simulink model "EPT"  (R2019b)
settings: Solver=FixedStepDiscrete  StartTime=0.0  StopTime=5  FixedStep=0.005  RelTol=1e-3  EnableMultiTasking=on
PreLoadFcn:
  | try, model_open; catch, disp('Error occurred while executing model pre-load callback: model_open.m'); disp('Please assure that the MATLAB working directory is set to the model directory before opening.'); end
InitFcn:
  | try, model_open; catch, end
undefined symbols (not defined in the file or in its folder): Bridge, GCM, H, ln, raptor_get_param_eval, raptor_get_safe_string, raptor_xcp_function
libraries: Raptor_lib x2810, simulink x374, hdlsllib x19
(part 18 of 45)

== system EPT/Foreground_TimeBase_5ms/CAN/CAN3_exec/DCDC/DCDC_RX_0x180XF45D  ==
  Trigger : TriggerPort  VariantControl=Variant  PortDimensions=1
  Constant : Constant  Value=0.1
  Constant1 : Constant  Value=-40
  Constant2 : Constant
  Convert_Byte2Data1 : Subsystem
  Convert_Byte2Data2 : Subsystem
  Convert_Byte2Data3 : Subsystem
  Demux : Demux  Outputs=8
  raptor_can_rxmsg : Raptor_lib/CAN/raptor_can_rxmsg  Commented=on  canDefinition=struct('dbcFile', 'DCDC_TDY_1Y_108_12 _V07.dbc','message', 'DCDC2EPT','comment', '','signals', {{'Output_Voltage','Output_Current','Internal_Temp','Status'}},'enabled', [ 1 1 1 1;],'canBus', '''CAN3''','messageID', [ 403174613;],'idMask', [ 536870911;],'payloadMask', [],'payloadValue', [],'period', [ 0;],'mailbox', '''''','queueSize', [ 1;],'label', [ 0;],'ver', [ 2;],'showID', [ 0;],'showRaw', [ 0;],'fill', [ 0;],'editID', [ 0;],'signalOrder', [ 2;])  canBus='CAN3'  mailbox=''  payloadMask=[]  payloadValue=[]  idMask=hex2dec('1FFFFFFF')  queueSize=1  showID=0  label=0  fill=0  id=403174613  showRaw=0  showAge=1  signalOrder=2  signalInfo={{struct('Name', 'Status','Startbit', [ 0;],'SignalSize', [ 8;],'ByteOrder', 'BigEndian','ValueType', 'UNSIGNED','Class', 'uint8','Signed', [ 0;],'Factor', [ 1;],'Offset', [ 0;],'Min', [ 0;],'Max', [ 0;],'Units', '','Comment', '','StartBit', [ 40;]),struct('Name', 'Output_Voltage','Startbit', [ 0;],'SignalSize', [ 16;],'ByteOrder', 'BigEndian','ValueType', 'UNSIGNED','Class', 'uint16','Signed', [ 0;],'Factor', [ 0.1;],'Offset', [ 0;],'Min', [ 0;],'Max', [ 0;],'Units', 'V','Comment', '','StartBit', [ 8;]),struct('Name', 'Output_Current','Startbit', [ 0;],'SignalSize', [ 16;],'ByteOrder', 'BigEndian','ValueType', 'UNSIGNED','Class', 'uint16','Signed', [ 0;],'Factor', [ 0.1;],'Offset', [ 0;],'Min', [ 0;],'Max', [ 0;],'Units', 'A','Comment', '','StartBit', [ 24;]),struct('Name', 'Internal_Temp','Startbit', [ 0;],'SignalSize', [ 8;],'ByteOrder', 'BigEndian','ValueType', 'UNSIGNED','Class', 'uint8','Signed', [ 0;],'Factor', [ 1;],'Offset', [ -40;],'Min', [ 0;],'Max', [ 0;],'Units', 'C','Comment', '','StartBit', [ 32;])}}
      settings: SourceProductName=Raptor
  raptor_can_rxraw : Raptor_lib/CAN/raptor_can_rxraw  canBus='CAN3'  extendedId=1  showAge=1  id=hex2dec('1806F4D5')  idMask=hex2dec('1FF0FFFF')  mailbox=''  queueSize=1
      settings: SourceProductName=Raptor
  raptor_data_def1 : Raptor_lib/Data Storage/raptor_data_def  dataName='Read_DCDC_Status'  initValue=0  dataType=uint8  storage=Volatile (RAM)  calVisible=on  calType=Measurement  calDispType=Number  calEnum={'False', 'True'}  calGain=1.0  calOffset=0  calMin=-inf  calMax=inf  calFormat='-1'  calUnit=''  calHelp=''  calAccess=1  calFunction=raptor_xcp_function(gcb)  calDispHeaders=off  calColHeaders={'Col1' 'Col2' 'Col3'}  calRowHeaders={'Row1' 'Row2' 'Row3'}
      settings: SourceProductName=Raptor
  raptor_data_def2 : Raptor_lib/Data Storage/raptor_data_def  dataName='Read_DCDC_Internal_Temp'  initValue=0  dataType=double  storage=Volatile (RAM)  calVisible=on  calType=Measurement  calDispType=Number  calEnum={'False', 'True'}  calGain=1.0  calOffset=0  calMin=-inf  calMax=inf  calFormat='-1'  calUnit=''  calHelp=''  calAccess=1  calFunction=raptor_xcp_function(gcb)  calDispHeaders=off  calColHeaders={'Col1' 'Col2' 'Col3'}  calRowHeaders={'Row1' 'Row2' 'Row3'}
      settings: SourceProductName=Raptor
  raptor_data_def3 : Raptor_lib/Data Storage/raptor_data_def  dataName='Read_DCDC_Output_Current'  initValue=0  dataType=double  storage=Volatile (RAM)  calVisible=on  calType=Measurement  calDispType=Number  calEnum={'False', 'True'}  calGain=1.0  calOffset=0  calMin=-inf  calMax=inf  calFormat='-1'  calUnit=''  calHelp=''  calAccess=1  calFunction=raptor_xcp_function(gcb)  calDispHeaders=off  calColHeaders={'Col1' 'Col2' 'Col3'}  calRowHeaders={'Row1' 'Row2' 'Row3'}
      settings: SourceProductName=Raptor
  raptor_data_def4 : Raptor_lib/Data Storage/raptor_data_def  dataName='Read_DCDC_Output_Voltage'  initValue=0  dataType=double  storage=Volatile (RAM)  calVisible=on  calType=Measurement  calDispType=Number  calEnum={'False', 'True'}  calGain=1.0  calOffset=0  calMin=-inf  calMax=inf  calFormat='-1'  calUnit=''  calHelp=''  calAccess=1  calFunction=raptor_xcp_function(gcb)  calDispHeaders=off  calColHeaders={'Col1' 'Col2' 'Col3'}  calRowHeaders={'Row1' 'Row2' 'Row3'}
      settings: SourceProductName=Raptor
  raptor_data_def5 : Raptor_lib/Data Storage/raptor_data_def  dataName='Rx0x180XF4D5_Age'  initValue=0  dataType=uint16  storage=Volatile (RAM)  calVisible=on  calType=Measurement  calDispType=Number  calEnum={'False', 'True'}  calGain=1.0  calOffset=0  calMin=-inf  calMax=inf  calFormat='-1'  calUnit=''  calHelp=''  calAccess=1  calFunction=raptor_xcp_function(gcb)  calDispHeaders=off  calColHeaders={'Col1' 'Col2' 'Col3'}  calRowHeaders={'Row1' 'Row2' 'Row3'}
      settings: SourceProductName=Raptor
  raptor_data_write1 : Raptor_lib/Data Storage/raptor_data_write  Commented=on  dataName='Read_DCDC_Status'  dataShape=Scalar  idxSource=Input Port  idxRow=1  idxCol=1
      settings: SourceProductName=Raptor
  raptor_data_write10 : Raptor_lib/Data Storage/raptor_data_write  Commented=on  dataName='Rx0x180XF4D5_Age'  dataShape=Scalar  idxSource=Input Port  idxRow=1  idxCol=1
      settings: SourceProductName=Raptor
  raptor_data_write2 : Raptor_lib/Data Storage/raptor_data_write  Commented=on  dataName='Read_DCDC_Internal_Temp'  dataShape=Scalar  idxSource=Input Port  idxRow=1  idxCol=1
      settings: SourceProductName=Raptor
  raptor_data_write3 : Raptor_lib/Data Storage/raptor_data_write  Commented=on  dataName='Read_DCDC_Output_Current'  dataShape=Scalar  idxSource=Input Port  idxRow=1  idxCol=1
      settings: SourceProductName=Raptor
  raptor_data_write4 : Raptor_lib/Data Storage/raptor_data_write  Commented=on  dataName='Read_DCDC_Output_Voltage'  dataShape=Scalar  idxSource=Input Port  idxRow=1  idxCol=1
      settings: SourceProductName=Raptor
  raptor_data_write5 : Raptor_lib/Data Storage/raptor_data_write  dataName='Rx0x180XF4D5_Age'  dataShape=Scalar  idxSource=Input Port  idxRow=1  idxCol=1
      settings: SourceProductName=Raptor
  raptor_data_write6 : Raptor_lib/Data Storage/raptor_data_write  dataName='Read_DCDC_Status'  dataShape=Scalar  idxSource=Input Port  idxRow=1  idxCol=1
      settings: SourceProductName=Raptor
  raptor_data_write7 : Raptor_lib/Data Storage/raptor_data_write  dataName='Read_DCDC_Internal_Temp'  dataShape=Scalar  idxSource=Input Port  idxRow=1  idxCol=1
      settings: SourceProductName=Raptor
  raptor_data_write8 : Raptor_lib/Data Storage/raptor_data_write  dataName='Read_DCDC_Output_Voltage'  dataShape=Scalar  idxSource=Input Port  idxRow=1  idxCol=1
      settings: SourceProductName=Raptor
  raptor_data_write9 : Raptor_lib/Data Storage/raptor_data_write  dataName='Read_DCDC_Output_Current'  dataShape=Scalar  idxSource=Input Port  idxRow=1  idxCol=1
      settings: SourceProductName=Raptor
  wires:
  raptor_can_rxmsg/3 -> raptor_data_write2/1
  raptor_can_rxmsg/4 -> raptor_data_write3/1
  raptor_can_rxmsg/1 -> raptor_data_write10/1
  raptor_can_rxraw/1 -> raptor_data_write5/1
  raptor_can_rxraw/5 -> Demux/1
  Demux/2 -> Convert_Byte2Data3/2(LowByte)
  Demux/1 -> Convert_Byte2Data3/1(HighByte)
  Demux/3 -> Convert_Byte2Data1/1(HighByte)
  Demux/4 -> Convert_Byte2Data1/2(LowByte)
  Constant/1 -> Convert_Byte2Data1/4(Factor), Convert_Byte2Data3/4(Factor)
  Demux/5 -> Convert_Byte2Data2/2(LowByte)
  Constant1/1 -> Convert_Byte2Data2/3(Offset)
  Constant2/1 -> Convert_Byte2Data2/4(Factor)
  raptor_can_rxmsg/5 -> raptor_data_write1/1
  raptor_can_rxmsg/2 -> raptor_data_write4/1
  Demux/6 -> raptor_data_write6/1
  Convert_Byte2Data2/1(Data) -> raptor_data_write7/1
  Convert_Byte2Data3/1(Data) -> raptor_data_write8/1
  Convert_Byte2Data1/1(Data) -> raptor_data_write9/1

== system EPT/Foreground_TimeBase_5ms/CAN/CAN3_exec/DCDC/DCDC_TX_0x180XD5F4 ==
  note: Notes:
      | 0: DC Output
      | 1: Shut Down Output
  Trigger : TriggerPort  TriggerType=falling  VariantControl=Variant  PortDimensions=1
  Constant : Constant  Value=8  OutDataTypeStr=uint8
  Constant1 : Constant  OutDataTypeStr=boolean
  Mux : Mux  Inputs=8
  raptor_adjustment : Raptor_lib/Data Storage/raptor_adjustment  paramName='Cal_DCDC_TxID'  nameSource=Parameter  initValue=hex2dec('1806D5F4')  dataType=uint32  storage=Calibration  calDispType=Number  calEnum={'False', 'True'}  calGain=1.0  calOffset=0.0  calMax=inf  calMin=-inf  calFormat='-1'  calUnit=''  calHelp=''  calAccess=1  calFunction=raptor_xcp_function(gcb)  calDispHeaders=off  calColHeaders={'Col1' 'Col2' 'Col3'}  calRowHeaders={'Row1' 'Row2' 'Row3'}
      settings: SourceProductName=Raptor
  raptor_can_txmsg : Raptor_lib/CAN/raptor_can_txmsg  Commented=on  canDefinition=struct('dbcFile', 'DCDC_TDY_1Y_108_12 _V07.dbc','message', 'EPT2DCDC','comment', '','signals', {{'DC_Control'}},'enabled', [ 1;],'canBus', '''CAN3''','messageID', [ 403166708;],'idMask', [ 536870911;],'payloadMask', [],'payloadValue', [],'period', [ 0;],'mailbox', '','queueSize', [ 1;],'label', [ 0;],'ver', [ 2;],'showID', [ 0;],'showRaw', [ 0;],'fill', [ 0;],'editID', [ 0;],'signalOrder', [ 1;])  canBus='CAN3'  queueSize=1  payloadMask=[]  payloadValue=[]  period=0  showID=0  label=0  idMask=hex2dec('1FFFFFFF')  fill=0  id=403166708  showRaw=0  signalOrder=1  signalInfo={{struct('Name', 'DC_Control','Startbit', [ 0;],'SignalSize', [ 8;],'ByteOrder', 'LittleEndian','ValueType', 'SIGNED','Class', 'int8','Signed', [ 1;],'Factor', [ 1;],'Offset', [ 0;],'Min', [ 0;],'Max', [ 0;],'Units', '','Comment', '','StartBit', [ 32;])}}
      settings: SourceProductName=Raptor
  raptor_can_txraw : Raptor_lib/CAN/raptor_can_txraw  canBus='CAN3'  queueSize=1  showIdTypePort=1  idTypeSelectValues=Standard|Extended  idTypeSelect=Standard
      settings: SourceProductName=Raptor
  raptor_data_def2 : Raptor_lib/Data Storage/raptor_data_def  dataName='Cmd_DC_Control'  initValue=1  dataType=uint8  storage=Volatile (RAM)  calVisible=on  calType=Measurement  calDispType=Number  calEnum={'False', 'True'}  calGain=1.0  calOffset=0  calMin=-inf  calMax=inf  calFormat='-1'  calUnit=''  calHelp=''  calAccess=1  calFunction=raptor_xcp_function(gcb)  calDispHeaders=off  calColHeaders={'Col1' 'Col2' 'Col3'}  calRowHeaders={'Row1' 'Row2' 'Row3'}
      settings: SourceProductName=Raptor
  raptor_data_read : Raptor_lib/Data Storage/raptor_data_read  Commented=on  dataName='Cmd_DC_Control'  dataShape=Scalar  idxSource=Input  idxRow=1  idxCol=1
      settings: SourceProductName=Raptor
  raptor_data_read1 : Raptor_lib/Data Storage/raptor_data_read  dataName='Cmd_DC_Control'  dataShape=Scalar  idxSource=Input  idxRow=1  idxCol=1
      settings: SourceProductName=Raptor
  wires:
  raptor_data_read/1 -> raptor_can_txmsg/1
  Constant/1 -> raptor_can_txraw/3
  Constant1/1 -> raptor_can_txraw/1
  Mux/1 -> raptor_can_txraw/4
  raptor_data_read1/1 -> Mux/5
  raptor_adjustment/1 -> raptor_can_txraw/2

== system EPT/Foreground_TimeBase_5ms/CAN/CAN3_exec/HyPer9_MCU/CountTrigger2 ==
  Counter : Inport
  Constant1 : Constant  Value=0
  Constant3 : Constant
  CycleTrigger : Subsystem
  Switch : Switch  Threshold=1
  Unit Delay1 : UnitDelay  SampleTime=-1  HasFrameUpgradeWarning=on
  Unit Delay2 : UnitDelay  SampleTime=-1  HasFrameUpgradeWarning=on
  Tirgger : Outport  VectorParamsAs1DForOutWhenUnconnected=off
  wires:
  Switch/1 -> Unit Delay1/1
  Constant3/1 -> Switch/3
  Constant1/1 -> Switch/1
  Counter/1 -> CycleTrigger/2(In2)
  CycleTrigger/1(Trigger) -> Switch/2, Unit Delay2/1
  Unit Delay1/1 -> CycleTrigger/1(In1)
  Unit Delay2/1 -> Tirgger/1

== system EPT/Foreground_TimeBase_5ms/CAN/CAN3_exec/HyPer9_MCU/RPDO1 ==
  note: Request for Mains State
      | 0: Ignored;
      | 1: Startup Request;
      | 2: Mains Check Request;
      | 3: Ignored;
      | 4: Pre-Charge Request;
      | 5: Ignored;
      | 6: Power Ready Request
      | 7: Alarm Request
      | 8: Power Ready Direct Request
      | 9: Power Ready External Precharge Request
  Trigger : TriggerPort  TriggerType=falling  VariantControl=Variant  PortDimensions=1
  Bit Shift : hdlsllib/Logic and Bit Operations/Bit Shift  mode=Shift Left Logical  N=3
  Byte1 : Subsystem
  Constant : Constant  Value=8  OutDataTypeStr=Inherit: Inherit via back propagation
  Constant1 : Constant  Value=hex2dec('200')  OutDataTypeStr=Inherit: Inherit via back propagation
  Constant2 : Constant  Value=32767  OutDataTypeStr=Inherit: Inherit via back propagation
  Constant3 : Constant  Value=32767  OutDataTypeStr=Inherit: Inherit via back propagation
  Constant4 : Constant  Value=32767  OutDataTypeStr=Inherit: Inherit via back propagation
  Convert_Data2Byte : Subsystem
  Convert_Data2Byte1 : Subsystem
  Convert_Data2Byte2 : Subsystem
  Data Type Conversion : DataTypeConversion  OutDataTypeStr=uint8
  Display : Display
  Gain : Gain  Gain=1/100
  Gain1 : Gain  Gain=1/100
  Gain2 : Gain  Gain=1/100
  IsPositive : simulink/Logic and Bit Operations/Compare To Zero  relop=>  OutDataTypeStr=boolean
  Mux : Mux  Inputs=8
  Request for Driver Output 1 in PWM Mode or in Current Mode : Constant  Value=0
  Request for Driver Output 2 in PWM Mode or in Current Mode : Constant  Value=0
  Request for Driver Output 3 in PWM Mode or in Current Mode : Constant  Value=0
  raptor_adjustment : Raptor_lib/Data Storage/raptor_adjustment  paramName='Cal_Request_for_Mains_State'  nameSource=Parameter  initValue=0.00  dataType=double  storage=Calibration  calDispType=Number  calEnum={'False', 'True'}  calGain=1.0  calOffset=0.0  calMax=9  calMin=-inf  calFormat='-1'  calUnit=''  calHelp=''  calAccess=1  calFunction=raptor_xcp_function(gcb)  calDispHeaders=off  calColHeaders={'Col1' 'Col2' 'Col3'}  calRowHeaders={'Row1' 'Row2' 'Row3'}
      settings: SourceProductName=Raptor
  raptor_can_txraw : Raptor_lib/CAN/raptor_can_txraw  canBus='CAN3'  queueSize=1  showIdTypePort=0  idTypeSelectValues=Standard|Extended  idTypeSelect=Standard
      settings: SourceProductName=Raptor
  raptor_override : Raptor_lib/Data Storage/raptor_override  paramName='Ovr_Request_for_Mains_State'  nameSource=Parameter  measurement=None  calDispType=Number  calEnum={'False', 'True'}  calGain=1.0  calOffset=0.0  calMax=inf  calMin=-inf  calFormat='-1'  calUnit=''  calHelp=''  calAccess=1  calFunction=[raptor_xcp_function(gcb) '|' raptor_get_param_eval(gcb, 'paramName') '_Override']
      settings: SourceProductName=Raptor
  wires:
  Mux/1 -> raptor_can_txraw/3
  Bit Shift/1 -> raptor_override/1
  IsPositive/1 -> Data Type Conversion/1
  raptor_adjustment/1 -> IsPositive/1
  Data Type Conversion/1 -> Bit Shift/1
  Byte1/1(Byte) -> Mux/2
  Convert_Data2Byte/1(LowByte) -> Mux/3
  Convert_Data2Byte/2(HighByte) -> Mux/4
  Convert_Data2Byte1/2(HighByte) -> Mux/6
  Convert_Data2Byte1/1(LowByte) -> Mux/5
  Convert_Data2Byte2/1(LowByte) -> Mux/7
  Convert_Data2Byte2/2(HighByte) -> Mux/8
  Constant2/1 -> Convert_Data2Byte/2(Factor)
  Request for Driver Output 1 in PWM Mode or in Current Mode/1 -> Gain/1
  Request for Driver Output 2 in PWM Mode or in Current Mode/1 -> Gain1/1
  Constant3/1 -> Convert_Data2Byte1/2(Factor)
  Constant4/1 -> Convert_Data2Byte2/2(Factor)
  Request for Driver Output 3 in PWM Mode or in Current Mode/1 -> Gain2/1
  Constant1/1 -> raptor_can_txraw/1
  Constant/1 -> raptor_can_txraw/2
  Gain/1 -> Convert_Data2Byte/1(Data)
  Gain1/1 -> Convert_Data2Byte1/1(Data)
  Gain2/1 -> Convert_Data2Byte2/1(Data)
  raptor_override/1 -> Display/1, Mux/1

== system EPT/Foreground_TimeBase_5ms/CAN/CAN3_exec/HyPer9_MCU/RPDO2 ==
  Trigger : TriggerPort  VariantControl=Variant  PortDimensions=1
  Byte5 : Subsystem
  Constant : Constant  Value=8  OutDataTypeStr=Inherit: Inherit via back propagation
  Constant1 : Constant  Value=hex2dec('300')  OutDataTypeStr=Inherit: Inherit via back propagation
  Constant2 : Constant  Value=32767  OutDataTypeStr=Inherit: Inherit via back propagation
  Constant3 : Constant  Value=255  OutDataTypeStr=Inherit: Inherit via back propagation
  Constant5 : Constant  Value=32767  OutDataTypeStr=double
  Convert_Data2Byte : Subsystem
  Convert_Data2Byte1 : Subsystem
  Convert_Data2Byte2 : Subsystem
  Display : Display
      settings: Format=hex (Stored Integer)
  Gain : Gain  Gain=1/100
  Gain1 : Gain  Gain=1/100
  Mux : Mux  Inputs=8
  raptor_adjustment : Raptor_lib/Data Storage/raptor_adjustment  paramName='Cal_Motor1_Speed_Limit'  nameSource=Parameter  initValue=0.00  dataType=double  storage=Calibration  calDispType=Number  calEnum={'False', 'True'}  calGain=1.0  calOffset=0.0  calMax=inf  calMin=-inf  calFormat='-1'  calUnit=''  calHelp=''  calAccess=1  calFunction=raptor_xcp_function(gcb)  calDispHeaders=off  calColHeaders={'Col1' 'Col2' 'Col3'}  calRowHeaders={'Row1' 'Row2' 'Row3'}
      settings: SourceProductName=Raptor
  raptor_adjustment1 : Raptor_lib/Data Storage/raptor_adjustment  paramName='Cal_Motor1_Torque_Reference'  nameSource=Parameter  initValue=0.00  dataType=double  storage=Calibration  calDispType=Number  calEnum={'False', 'True'}  calGain=1.0  calOffset=0.0  calMax=inf  calMin=-inf  calFormat='-1'  calUnit=''  calHelp=''  calAccess=1  calFunction=raptor_xcp_function(gcb)  calDispHeaders=off  calColHeaders={'Col1' 'Col2' 'Col3'}  calRowHeaders={'Row1' 'Row2' 'Row3'}
      settings: SourceProductName=Raptor
  raptor_adjustment2 : Raptor_lib/Data Storage/raptor_adjustment  paramName='Cal_Motor1_Droop_Rate'  nameSource=Parameter  initValue=25  dataType=double  storage=Calibration  calDispType=Number  calEnum={'False', 'True'}  calGain=1.0  calOffset=0.0  calMax=inf  calMin=-inf  calFormat='-1'  calUnit=''  calHelp=''  calAccess=1  calFunction=raptor_xcp_function(gcb)  calDispHeaders=off  calColHeaders={'Col1' 'Col2' 'Col3'}  calRowHeaders={'Row1' 'Row2' 'Row3'}
      settings: SourceProductName=Raptor
  raptor_can_txraw : Raptor_lib/CAN/raptor_can_txraw  canBus='CAN3'  queueSize=1  showIdTypePort=0  idTypeSelectValues=Standard|Extended  idTypeSelect=Standard
      settings: SourceProductName=Raptor
  wires:
  Constant/1 -> raptor_can_txraw/2
  Constant1/1 -> raptor_can_txraw/1
  Constant3/1 -> Convert_Data2Byte2/2(Factor)
  raptor_adjustment2/1 -> Gain/1
  raptor_adjustment1/1 -> Gain1/1
  Convert_Data2Byte2/1(LowByte) -> Mux/5, Display/1
  Convert_Data2Byte1/2(HighByte) -> Mux/4
  Convert_Data2Byte1/1(LowByte) -> Mux/3
  Mux/1 -> raptor_can_txraw/3
  Convert_Data2Byte/1(LowByte) -> Mux/1
  Convert_Data2Byte/2(HighByte) -> Mux/2
  Constant2/1 -> Convert_Data2Byte1/2(Factor)
  Byte5/1(Byte) -> Mux/6
  Gain/1 -> Convert_Data2Byte2/1(Data)
  Gain1/1 -> Convert_Data2Byte1/1(Data)
  raptor_adjustment/1 -> Convert_Data2Byte/1(Data)

== system EPT/Foreground_TimeBase_5ms/CAN/CAN3_exec/HyPer9_MCU/RPDO3 ==
  Trigger : TriggerPort  VariantControl=Variant  PortDimensions=1
  Byte5 : Subsystem
  Constant : Constant  Value=8  OutDataTypeStr=Inherit: Inherit via back propagation
  Constant1 : Constant  Value=hex2dec('400')  OutDataTypeStr=Inherit: Inherit via back propagation
  Constant2 : Constant  Value=32767  OutDataTypeStr=Inherit: Inherit via back propagation
  Constant3 : Constant  Value=32767  OutDataTypeStr=Inherit: Inherit via back propagation
  Constant5 : Constant  Value=32767  OutDataTypeStr=double
  Convert_Data2Byte : Subsystem
  Convert_Data2Byte1 : Subsystem
  Convert_Data2Byte2 : Subsystem
  Display : Display
      settings: Format=hex (Stored Integer)
  Gain : Gain  Gain=1/100
  Gain1 : Gain  Gain=1/100
  Mux : Mux  Inputs=8
  raptor_adjustment : Raptor_lib/Data Storage/raptor_adjustment  paramName='Cal_Motor2_Speed_Limit'  nameSource=Parameter  initValue=0.00  dataType=double  storage=Calibration  calDispType=Number  calEnum={'False', 'True'}  calGain=1.0  calOffset=0.0  calMax=inf  calMin=-inf  calFormat='-1'  calUnit=''  calHelp=''  calAccess=1  calFunction=raptor_xcp_function(gcb)  calDispHeaders=off  calColHeaders={'Col1' 'Col2' 'Col3'}  calRowHeaders={'Row1' 'Row2' 'Row3'}
      settings: SourceProductName=Raptor
  raptor_adjustment1 : Raptor_lib/Data Storage/raptor_adjustment  paramName='Cal_Motor2_Torque_Reference'  nameSource=Parameter  initValue=0.00  dataType=double  storage=Calibration  calDispType=Number  calEnum={'False', 'True'}  calGain=1.0  calOffset=0.0  calMax=inf  calMin=-inf  calFormat='-1'  calUnit=''  calHelp=''  calAccess=1  calFunction=raptor_xcp_function(gcb)  calDispHeaders=off  calColHeaders={'Col1' 'Col2' 'Col3'}  calRowHeaders={'Row1' 'Row2' 'Row3'}
      settings: SourceProductName=Raptor
  raptor_adjustment2 : Raptor_lib/Data Storage/raptor_adjustment  paramName='Cal_Motor2_Droop_Rate'  nameSource=Parameter  initValue=25  dataType=double  storage=Calibration  calDispType=Number  calEnum={'False', 'True'}  calGain=1.0  calOffset=0.0  calMax=inf  calMin=-inf  calFormat='-1'  calUnit=''  calHelp=''  calAccess=1  calFunction=raptor_xcp_function(gcb)  calDispHeaders=off  calColHeaders={'Col1' 'Col2' 'Col3'}  calRowHeaders={'Row1' 'Row2' 'Row3'}
      settings: SourceProductName=Raptor
  raptor_can_txraw : Raptor_lib/CAN/raptor_can_txraw  canBus='CAN3'  queueSize=1  showIdTypePort=0  idTypeSelectValues=Standard|Extended  idTypeSelect=Standard
      settings: SourceProductName=Raptor
  wires:
  Byte5/1(Byte) -> Mux/6
  Constant2/1 -> Convert_Data2Byte1/2(Factor)
  Convert_Data2Byte/2(HighByte) -> Mux/2
  Convert_Data2Byte/1(LowByte) -> Mux/1
  Mux/1 -> raptor_can_txraw/3
  Convert_Data2Byte1/1(LowByte) -> Mux/3
  Convert_Data2Byte1/2(HighByte) -> Mux/4
  raptor_adjustment1/1 -> Gain1/1
  Constant1/1 -> raptor_can_txraw/1
  Constant/1 -> raptor_can_txraw/2
  raptor_adjustment2/1 -> Gain/1
  Constant3/1 -> Convert_Data2Byte2/2(Factor)
  Convert_Data2Byte2/1(LowByte) -> Mux/5, Display/1
  Gain/1 -> Convert_Data2Byte2/1(Data)
  Gain1/1 -> Convert_Data2Byte1/1(Data)
  raptor_adjustment/1 -> Convert_Data2Byte/1(Data)

== system EPT/Foreground_TimeBase_5ms/CAN/CAN3_exec/HyPer9_MCU/RPDO4 ==
  Trigger : TriggerPort  TriggerType=falling  VariantControl=Variant  PortDimensions=1
  Constant : Constant  Value=8  OutDataTypeStr=Inherit: Inherit via back propagation
  Constant1 : Constant  Value=hex2dec('500')  OutDataTypeStr=Inherit: Inherit via back propagation
  Convert_Data2Byte : Subsystem
  Convert_Data2Byte1 : Subsystem
  Mux : Mux  Inputs=8
  raptor_adjustment : Raptor_lib/Data Storage/raptor_adjustment  paramName='Cal_Battery_Charge_Current_Limit'  nameSource=Parameter  initValue=0.00  dataType=double  storage=Calibration  calDispType=Number  calEnum={'False', 'True'}  calGain=1.0  calOffset=0.0  calMax=inf  calMin=-inf  calFormat='-1'  calUnit=''  calHelp=''  calAccess=1  calFunction=raptor_xcp_function(gcb)  calDispHeaders=off  calColHeaders={'Col1' 'Col2' 'Col3'}  calRowHeaders={'Row1' 'Row2' 'Row3'}
      settings: SourceProductName=Raptor
  raptor_adjustment1 : Raptor_lib/Data Storage/raptor_adjustment  paramName='Cal_Battery_Discharge_Current_Limit'  nameSource=Parameter  initValue=0.00  dataType=double  storage=Calibration  calDispType=Number  calEnum={'False', 'True'}  calGain=1.0  calOffset=0.0  calMax=inf  calMin=-inf  calFormat='-1'  calUnit=''  calHelp=''  calAccess=1  calFunction=raptor_xcp_function(gcb)  calDispHeaders=off  calColHeaders={'Col1' 'Col2' 'Col3'}  calRowHeaders={'Row1' 'Row2' 'Row3'}
      settings: SourceProductName=Raptor
  raptor_can_txraw : Raptor_lib/CAN/raptor_can_txraw  canBus='CAN3'  queueSize=1  showIdTypePort=0  idTypeSelectValues=Standard|Extended  idTypeSelect=Standard
      settings: SourceProductName=Raptor
  wires:
  Mux/1 -> raptor_can_txraw/3
  Convert_Data2Byte1/1(LowByte) -> Mux/3
  Convert_Data2Byte1/2(HighByte) -> Mux/4
  raptor_adjustment1/1 -> Convert_Data2Byte1/1(Data)
  Constant1/1 -> raptor_can_txraw/1
  Constant/1 -> raptor_can_txraw/2
  raptor_adjustment/1 -> Convert_Data2Byte/1(Data)
  Convert_Data2Byte/2(HighByte) -> Mux/2
  Convert_Data2Byte/1(LowByte) -> Mux/1

== system EPT/Foreground_TimeBase_5ms/CAN/CAN3_exec/HyPer9_MCU/TPDO1 ==
  Trigger : TriggerPort  TriggerType=falling  VariantControl=Variant  PortDimensions=1
  Constant : Constant  Value=0.1  OutDataTypeStr=double
  Constant1 : Constant  Value=0.1  OutDataTypeStr=double
  Constant2 : Constant  Value=0.1  OutDataTypeStr=double
  Convert_Byte2Data : Subsystem
  Convert_Byte2Data1 : Subsystem
  Convert_Byte2Data2 : Subsystem
  Demux : Demux  Outputs=8
  "Mains State " : Subsystem
  Mux : Mux  Inputs=7
  raptor_can_rxraw : Raptor_lib/CAN/raptor_can_rxraw  canBus='CAN3'  extendedId=0  showAge=1  id=hex2dec('180')  idMask=hex2dec('1FFFFFFF')  mailbox=''  queueSize=1
      settings: SourceProductName=Raptor
  raptor_measurement : Raptor_lib/Data Storage/raptor_measurement  paramName='Meas_Mains_State'  nameSource=Parameter  calDispType=Number  calEnum={'False', 'True'}  calGain=1.0  calOffset=0.0  calMax=inf  calMin=-inf  calFormat='-1'  calUnit=''  calHelp=''  calAccess=1  calFunction=raptor_xcp_function(gcb)  calVisible=on
      settings: SourceProductName=Raptor
  raptor_measurement1 : Raptor_lib/Data Storage/raptor_measurement  paramName='Meas_Fault_Code'  nameSource=Parameter  calDispType=Number  calEnum={'False', 'True'}  calGain=1.0  calOffset=0.0  calMax=inf  calMin=-inf  calFormat='-1'  calUnit=''  calHelp=''  calAccess=1  calFunction=raptor_xcp_function(gcb)  calVisible=on
      settings: SourceProductName=Raptor
  raptor_measurement2 : Raptor_lib/Data Storage/raptor_measurement  paramName='Meas_DC_Bus_Voltage'  nameSource=Parameter  calDispType=Number  calEnum={'False', 'True'}  calGain=1.0  calOffset=0.0  calMax=inf  calMin=-inf  calFormat='-1'  calUnit=''  calHelp=''  calAccess=1  calFunction=raptor_xcp_function(gcb)  calVisible=on
      settings: SourceProductName=Raptor
  raptor_measurement3 : Raptor_lib/Data Storage/raptor_measurement  paramName='Meas_DC_Bus_Current'  nameSource=Parameter  calDispType=Number  calEnum={'False', 'True'}  calGain=1.0  calOffset=0.0  calMax=inf  calMin=-inf  calFormat='-1'  calUnit=''  calHelp=''  calAccess=1  calFunction=raptor_xcp_function(gcb)  calVisible=on
      settings: SourceProductName=Raptor
  raptor_measurement4 : Raptor_lib/Data Storage/raptor_measurement  paramName='Meas_Power_Battery_Voltage'  nameSource=Parameter  calDispType=Number  calEnum={'False', 'True'}  calGain=1.0  calOffset=0.0  calMax=inf  calMin=-inf  calFormat='-1'  calUnit=''  calHelp=''  calAccess=1  calFunction=raptor_xcp_function(gcb)  calVisible=on
      settings: SourceProductName=Raptor
  raptor_measurement5 : Raptor_lib/Data Storage/raptor_measurement  paramName='Meas_Mains_State_Value'  nameSource=Parameter  calDispType=Number  calEnum={'False', 'True'}  calGain=1.0  calOffset=0.0  calMax=inf  calMin=-inf  calFormat='-1'  calUnit=''  calHelp=''  calAccess=1  calFunction=raptor_xcp_function(gcb)  calVisible=on
      settings: SourceProductName=Raptor
  wires:
  raptor_can_rxraw/5 -> Demux/1
  Demux/1 -> raptor_measurement5/1, "Mains State "/1(Byte)
  Demux/2 -> raptor_measurement1/1
  Demux/3 -> Convert_Byte2Data/1(LowByte)
  Demux/4 -> Convert_Byte2Data/2(HighByte)
  Convert_Byte2Data/1(Data) -> raptor_measurement2/1
  Convert_Byte2Data1/1(Data) -> raptor_measurement3/1
  Demux/6 -> Convert_Byte2Data1/2(HighByte)
  Demux/5 -> Convert_Byte2Data1/1(LowByte)
  Demux/7 -> Convert_Byte2Data2/1(LowByte)
  Demux/8 -> Convert_Byte2Data2/2(HighByte)
  Convert_Byte2Data2/1(Data) -> raptor_measurement4/1
  Constant/1 -> Convert_Byte2Data/4(Factor)
  Constant1/1 -> Convert_Byte2Data1/4(Factor)
  Constant2/1 -> Convert_Byte2Data2/4(Factor)
  "Mains State "/1(Startup) -> Mux/1
  "Mains State "/2(Mains Checking) -> Mux/2
  "Mains State "/3(Mains OK) -> Mux/3
  "Mains State "/4(Pre-Charging) -> Mux/4
  "Mains State "/5(Pre-Charge Done) -> Mux/5
  "Mains State "/6("Power Ready ") -> Mux/6
  "Mains State "/7("Alarmed ") -> Mux/7
  Mux/1 -> raptor_measurement/1

== system EPT/Foreground_TimeBase_5ms/CAN/CAN3_exec/HyPer9_MCU/TPDO2 ==
  Trigger : TriggerPort  VariantControl=Variant  PortDimensions=1
  Constant{,1..3} (4 alike) : Constant  Value=0.001  OutDataTypeStr=double
  Convert_Byte2Data : Subsystem
  Convert_Byte2Data1 : Subsystem
  Convert_Byte2Data2 : Subsystem
  Convert_Byte2Data3 : Subsystem
  Demux : Demux  Outputs=8
  raptor_can_rxraw : Raptor_lib/CAN/raptor_can_rxraw  canBus='CAN3'  extendedId=0  showAge=1  id=hex2dec('280')  idMask=hex2dec('1FFFFFFF')  mailbox=''  queueSize=1
      settings: SourceProductName=Raptor
  raptor_measurement : Raptor_lib/Data Storage/raptor_measurement  paramName='Meas_Analog_Input1'  nameSource=Parameter  calDispType=Number  calEnum={'False', 'True'}  calGain=1.0  calOffset=0.0  calMax=inf  calMin=-inf  calFormat='-1'  calUnit=''  calHelp=''  calAccess=1  calFunction=raptor_xcp_function(gcb)  calVisible=on
      settings: SourceProductName=Raptor
  raptor_measurement1 : Raptor_lib/Data Storage/raptor_measurement  paramName='Meas_Analog_Input2'  nameSource=Parameter  calDispType=Number  calEnum={'False', 'True'}  calGain=1.0  calOffset=0.0  calMax=inf  calMin=-inf  calFormat='-1'  calUnit=''  calHelp=''  calAccess=1  calFunction=raptor_xcp_function(gcb)  calVisible=on
      settings: SourceProductName=Raptor
  raptor_measurement2 : Raptor_lib/Data Storage/raptor_measurement  paramName='Meas_Analog_Input3'  nameSource=Parameter  calDispType=Number  calEnum={'False', 'True'}  calGain=1.0  calOffset=0.0  calMax=inf  calMin=-inf  calFormat='-1'  calUnit=''  calHelp=''  calAccess=1  calFunction=raptor_xcp_function(gcb)  calVisible=on
      settings: SourceProductName=Raptor
  raptor_measurement3 : Raptor_lib/Data Storage/raptor_measurement  paramName='Meas_Analog_Input4'  nameSource=Parameter  calDispType=Number  calEnum={'False', 'True'}  calGain=1.0  calOffset=0.0  calMax=inf  calMin=-inf  calFormat='-1'  calUnit=''  calHelp=''  calAccess=1  calFunction=raptor_xcp_function(gcb)  calVisible=on
      settings: SourceProductName=Raptor
  wires:
  Constant2/1 -> Convert_Byte2Data2/4(Factor)
  Constant1/1 -> Convert_Byte2Data1/4(Factor)
  Constant/1 -> Convert_Byte2Data/4(Factor)
  Convert_Byte2Data2/1(Data) -> raptor_measurement2/1
  Demux/6 -> Convert_Byte2Data2/2(HighByte)
  Demux/5 -> Convert_Byte2Data2/1(LowByte)
  Demux/3 -> Convert_Byte2Data1/1(LowByte)
  Demux/4 -> Convert_Byte2Data1/2(HighByte)
  Convert_Byte2Data1/1(Data) -> raptor_measurement1/1
  Convert_Byte2Data/1(Data) -> raptor_measurement/1
  Demux/2 -> Convert_Byte2Data/2(HighByte)
  Demux/1 -> Convert_Byte2Data/1(LowByte)
  raptor_can_rxraw/5 -> Demux/1
  Demux/7 -> Convert_Byte2Data3/1(LowByte)
  Demux/8 -> Convert_Byte2Data3/2(HighByte)
  Convert_Byte2Data3/1(Data) -> raptor_measurement3/1
  Constant3/1 -> Convert_Byte2Data3/4(Factor)

== system EPT/Foreground_TimeBase_5ms/CAN/CAN3_exec/HyPer9_MCU/TPDO3 ==
  Trigger : TriggerPort  TriggerType=falling  VariantControl=Variant  PortDimensions=1
  Byte6 : Subsystem
  Byte7 : Subsystem
  Constant : Constant  Value=0.001  OutDataTypeStr=double
  Constant1 : Constant  Value=0.001  OutDataTypeStr=double
  Convert_Byte2Data : Subsystem
  Convert_Byte2Data1 : Subsystem
  Demux : Demux  Outputs=8
  Digital Input 1 to 8 - State : Subsystem
  Digital Input 9 to 16 - State : Subsystem
  Mux : Mux  Inputs=8
  Mux1 : Mux  Inputs=8
  raptor_can_rxraw : Raptor_lib/CAN/raptor_can_rxraw  canBus='CAN3'  extendedId=0  showAge=1  id=hex2dec('380')  idMask=hex2dec('1FFFFFFF')  mailbox=''  queueSize=1
      settings: SourceProductName=Raptor
  raptor_measurement : Raptor_lib/Data Storage/raptor_measurement  paramName='Meas_Analog_Input5'  nameSource=Parameter  calDispType=Number  calEnum={'False', 'True'}  calGain=1.0  calOffset=0.0  calMax=inf  calMin=-inf  calFormat='-1'  calUnit=''  calHelp=''  calAccess=1  calFunction=raptor_xcp_function(gcb)  calVisible=on
      settings: SourceProductName=Raptor
  raptor_measurement1 : Raptor_lib/Data Storage/raptor_measurement  paramName='Meas_Analog_Input6'  nameSource=Parameter  calDispType=Number  calEnum={'False', 'True'}  calGain=1.0  calOffset=0.0  calMax=inf  calMin=-inf  calFormat='-1'  calUnit=''  calHelp=''  calAccess=1  calFunction=raptor_xcp_function(gcb)  calVisible=on
      settings: SourceProductName=Raptor
  raptor_measurement2 : Raptor_lib/Data Storage/raptor_measurement  paramName='Meas_Digital_Input1_8'  nameSource=Parameter  calDispType=Number  calEnum={'False', 'True'}  calGain=1.0  calOffset=0.0  calMax=inf  calMin=-inf  calFormat='-1'  calUnit=''  calHelp=''  calAccess=1  calFunction=raptor_xcp_function(gcb)  calVisible=on
      settings: SourceProductName=Raptor
  raptor_measurement3 : Raptor_lib/Data Storage/raptor_measurement  paramName='Meas_Digital_Input9_16'  nameSource=Parameter  calDispType=Number  calEnum={'False', 'True'}  calGain=1.0  calOffset=0.0  calMax=inf  calMin=-inf  calFormat='-1'  calUnit=''  calHelp=''  calAccess=1  calFunction=raptor_xcp_function(gcb)  calVisible=on
      settings: SourceProductName=Raptor
  wires:
  raptor_can_rxraw/5 -> Demux/1
  Demux/1 -> Convert_Byte2Data/1(LowByte)
  Demux/2 -> Convert_Byte2Data/2(HighByte)
  Convert_Byte2Data/1(Data) -> raptor_measurement/1
  Convert_Byte2Data1/1(Data) -> raptor_measurement1/1
  Demux/4 -> Convert_Byte2Data1/2(HighByte)
  Demux/3 -> Convert_Byte2Data1/1(LowByte)
  Constant/1 -> Convert_Byte2Data/4(Factor)
  Constant1/1 -> Convert_Byte2Data1/4(Factor)
  Demux/5 -> Digital Input 1 to 8 - State/1(Byte)
  Demux/6 -> Digital Input 9 to 16 - State/1(Byte)
  Demux/7 -> Byte6/1(Byte)
  Demux/8 -> Byte7/1(Byte)
  Digital Input 1 to 8 - State/2(Digital Input 2 State) -> Mux/2
  Digital Input 1 to 8 - State/3(Digital Input 3 State) -> Mux/3
  Digital Input 1 to 8 - State/1(Digital Input 1 State) -> Mux/1
  Digital Input 1 to 8 - State/4(Digital Input 4 State) -> Mux/4
  Digital Input 1 to 8 - State/5(Digital Input 5 State) -> Mux/5
  Digital Input 1 to 8 - State/6(Digital Input 6 State) -> Mux/6
  Digital Input 1 to 8 - State/7(Digital Input 7 State) -> Mux/7
  Digital Input 1 to 8 - State/8(Digital Input 8 State) -> Mux/8
  Mux/1 -> raptor_measurement2/1
  Mux1/1 -> raptor_measurement3/1
  Digital Input 9 to 16 - State/8(Digital Input 16 State) -> Mux1/8
  Digital Input 9 to 16 - State/7(Digital Input 15 State) -> Mux1/7
  Digital Input 9 to 16 - State/6(Digital Input 14 State) -> Mux1/6
  Digital Input 9 to 16 - State/5(Digital Input 13 State) -> Mux1/5
  Digital Input 9 to 16 - State/4(Digital Input 12 State) -> Mux1/4
  Digital Input 9 to 16 - State/1(Digital Input 9 State) -> Mux1/1
  Digital Input 9 to 16 - State/3(Digital Input 11 State) -> Mux1/3
  Digital Input 9 to 16 - State/2(Digital Input 10 State) -> Mux1/2

== system EPT/Foreground_TimeBase_5ms/CAN/CAN3_exec/HyPer9_MCU/TPDO4 ==
  note: Motor 1 - State
      | 0: Not yet defined;
      | 1: Disabled → PWM Outputs Off;
      | 2: Fluxed → PWM Outputs On and motor fluxed;
      | 3: Normal Operating → speed/torque reference enabled;
      | 4: Emergency Stop → the emergency stop rates are applied until 0 speed;
      | 5: Safe Stop → the safe stop rates are applied;
      | 6: Speed Limit → the speed is limited to the value set by user following its embedded rate;
  note: Motor 1 - Control Mode
      | 1 = Speed Mode
      | 2 = Torque Mode
      | 0 = No Request
  Trigger : TriggerPort  VariantControl=Variant  PortDimensions=1
  Byte6 : Subsystem
  Constant1 : Constant  Value=-100/372768  OutDataTypeStr=double
  Constant2 : Constant  Value=-40  OutDataTypeStr=double
  Constant3 : Constant  Value=-40  OutDataTypeStr=double
  Convert_Byte2Data : Subsystem
  Convert_Byte2Data1 : Subsystem
  Convert_Byte2Data2 : Subsystem
  Convert_Byte2Data3 : Subsystem
  Demux : Demux  Outputs=8
  Motor 1 - State : Subsystem
  raptor_can_rxraw : Raptor_lib/CAN/raptor_can_rxraw  canBus='CAN3'  extendedId=0  showAge=1  id=hex2dec('480')  idMask=hex2dec('1FFFFFFF')  mailbox=''  queueSize=1
      settings: SourceProductName=Raptor
  raptor_measurement1 : Raptor_lib/Data Storage/raptor_measurement  paramName='Meas_Motor1_Temperature'  nameSource=Parameter  calDispType=Number  calEnum={'False', 'True'}  calGain=1.0  calOffset=0.0  calMax=inf  calMin=-inf  calFormat='-1'  calUnit=''  calHelp=''  calAccess=1  calFunction=raptor_xcp_function(gcb)  calVisible=on
      settings: SourceProductName=Raptor
  raptor_measurement10 : Raptor_lib/Data Storage/raptor_measurement  paramName='Meas_Motor1_Safe_Stop'  nameSource=Parameter  calDispType=Number  calEnum={'False', 'True'}  calGain=1.0  calOffset=0.0  calMax=inf  calMin=-inf  calFormat='-1'  calUnit=''  calHelp=''  calAccess=1  calFunction=raptor_xcp_function(gcb)  calVisible=on
      settings: SourceProductName=Raptor
  raptor_measurement11 : Raptor_lib/Data Storage/raptor_measurement  paramName='Meas_Motor1_Actual_Speed'  nameSource=Parameter  calDispType=Number  calEnum={'False', 'True'}  calGain=1.0  calOffset=0.0  calMax=inf  calMin=-inf  calFormat='-1'  calUnit=''  calHelp=''  calAccess=1  calFunction=raptor_xcp_function(gcb)  calVisible=on
      settings: SourceProductName=Raptor
  raptor_measurement2 : Raptor_lib/Data Storage/raptor_measurement  paramName='Meas_Inverter1_Temperature'  nameSource=Parameter  calDispType=Number  calEnum={'False', 'True'}  calGain=1.0  calOffset=0.0  calMax=inf  calMin=-inf  calFormat='-1'  calUnit=''  calHelp=''  calAccess=1  calFunction=raptor_xcp_function(gcb)  calVisible=on
      settings: SourceProductName=Raptor
  raptor_measurement3 : Raptor_lib/Data Storage/raptor_measurement  paramName='Meas_Motor1_Actual_Relative_Torque'  nameSource=Parameter  calDispType=Number  calEnum={'False', 'True'}  calGain=1.0  calOffset=0.0  calMax=inf  calMin=-inf  calFormat='-1'  calUnit=''  calHelp=''  calAccess=1  calFunction=raptor_xcp_function(gcb)  calVisible=on
      settings: SourceProductName=Raptor
  raptor_measurement4 : Raptor_lib/Data Storage/raptor_measurement  paramName='Meas_Motor1_Crl_Mode'  nameSource=Parameter  calDispType=Number  calEnum={'False', 'True'}  calGain=1.0  calOffset=0.0  calMax=inf  calMin=-inf  calFormat='-1'  calUnit=''  calHelp=''  calAccess=1  calFunction=raptor_xcp_function(gcb)  calVisible=on
      settings: SourceProductName=Raptor
  raptor_measurement5 : Raptor_lib/Data Storage/raptor_measurement  paramName='Meas_Motor1_SPD_Limit'  nameSource=Parameter  calDispType=Number  calEnum={'False', 'True'}  calGain=1.0  calOffset=0.0  calMax=inf  calMin=-inf  calFormat='-1'  calUnit=''  calHelp=''  calAccess=1  calFunction=raptor_xcp_function(gcb)  calVisible=on
      settings: SourceProductName=Raptor
  raptor_measurement6 : Raptor_lib/Data Storage/raptor_measurement  paramName='Meas_Motor1_State'  nameSource=Parameter  calDispType=Number  calEnum={'False', 'True'}  calGain=1.0  calOffset=0.0  calMax=inf  calMin=-inf  calFormat='-1'  calUnit=''  calHelp=''  calAccess=1  calFunction=raptor_xcp_function(gcb)  calVisible=on
      settings: SourceProductName=Raptor
  raptor_measurement7 : Raptor_lib/Data Storage/raptor_measurement  paramName='Meas_Motor1_PWM_Output'  nameSource=Parameter  calDispType=Number  calEnum={'False', 'True'}  calGain=1.0  calOffset=0.0  calMax=inf  calMin=-inf  calFormat='-1'  calUnit=''  calHelp=''  calAccess=1  calFunction=raptor_xcp_function(gcb)  calVisible=on
      settings: SourceProductName=Raptor
  raptor_measurement8 : Raptor_lib/Data Storage/raptor_measurement  paramName='Meas_Motor1_REF_SPD_TRQ'  nameSource=Parameter  calDispType=Number  calEnum={'False', 'True'}  calGain=1.0  calOffset=0.0  calMax=inf  calMin=-inf  calFormat='-1'  calUnit=''  calHelp=''  calAccess=1  calFunction=raptor_xcp_function(gcb)  calVisible=on
      settings: SourceProductName=Raptor
  raptor_measurement9 : Raptor_lib/Data Storage/raptor_measurement  paramName='Meas_Motor1_Emergency_Stop'  nameSource=Parameter  calDispType=Number  calEnum={'False', 'True'}  calGain=1.0  calOffset=0.0  calMax=inf  calMin=-inf  calFormat='-1'  calUnit=''  calHelp=''  calAccess=1  calFunction=raptor_xcp_function(gcb)  calVisible=on
      settings: SourceProductName=Raptor
  wires:
  Demux/8 -> Motor 1 - State/1(Byte)
  Demux/7 -> Byte6/1(Byte)
  Demux/6 -> Convert_Byte2Data3/2(LowByte)
  Demux/5 -> Convert_Byte2Data2/2(LowByte)
  Constant1/1 -> Convert_Byte2Data1/4(Factor)
  Demux/3 -> Convert_Byte2Data1/1(LowByte)
  Demux/4 -> Convert_Byte2Data1/2(HighByte)
  Convert_Byte2Data1/1(Data) -> raptor_measurement3/1
  Convert_Byte2Data/1(Data) -> raptor_measurement11/1
  Demux/2 -> Convert_Byte2Data/2(HighByte)
  Demux/1 -> Convert_Byte2Data/1(LowByte)
  raptor_can_rxraw/5 -> Demux/1
  Convert_Byte2Data2/1(Data) -> raptor_measurement1/1
  Constant2/1 -> Convert_Byte2Data2/1(Offset)
  Convert_Byte2Data3/1(Data) -> raptor_measurement2/1
  Constant3/1 -> Convert_Byte2Data3/1(Offset)
  Byte6/1(Motor 1 - Control Mode) -> raptor_measurement4/1
  Motor 1 - State/1(Motor 1 - State) -> raptor_measurement6/1
  Byte6/6(Motor 1 - Speed Limit) -> raptor_measurement5/1
  Byte6/2(Motor 1 - PWM Output) -> raptor_measurement7/1
  Byte6/3(Motor 1 - Reference Speed/Torque) -> raptor_measurement8/1
  Byte6/4(Motor 1 - Emergency Stop) -> raptor_measurement9/1
  Byte6/5(Motor 1 - Safe Stop) -> raptor_measurement10/1

== system EPT/Foreground_TimeBase_5ms/CAN/CAN3_exec/HyPer9_MCU/TPDO5 ==
  Trigger : TriggerPort  TriggerType=falling  VariantControl=Variant  PortDimensions=1
  Byte6 : Subsystem
  Byte7 : Subsystem
  Constant1 : Constant  Value=-100/32768  OutDataTypeStr=double
  Constant2 : Constant  Value=-40  OutDataTypeStr=double
  Constant3 : Constant  Value=-40  OutDataTypeStr=double
  Convert_Byte2Data : Subsystem
  Convert_Byte2Data1 : Subsystem
  Convert_Byte2Data2 : Subsystem
  Convert_Byte2Data3 : Subsystem
  Demux : Demux  Outputs=8
  raptor_can_rxraw : Raptor_lib/CAN/raptor_can_rxraw  canBus='CAN3'  extendedId=0  showAge=1  id=hex2dec('680')  idMask=hex2dec('1FFFFFFF')  mailbox=''  queueSize=1
      settings: SourceProductName=Raptor
  raptor_measurement1 : Raptor_lib/Data Storage/raptor_measurement  paramName='Meas_Motor2_Temperature'  nameSource=Parameter  calDispType=Number  calEnum={'False', 'True'}  calGain=1.0  calOffset=0.0  calMax=inf  calMin=-inf  calFormat='-1'  calUnit=''  calHelp=''  calAccess=1  calFunction=raptor_xcp_function(gcb)  calVisible=on
      settings: SourceProductName=Raptor
  raptor_measurement10 : Raptor_lib/Data Storage/raptor_measurement  paramName='Meas_Motor2_Safe_Stop'  nameSource=Parameter  calDispType=Number  calEnum={'False', 'True'}  calGain=1.0  calOffset=0.0  calMax=inf  calMin=-inf  calFormat='-1'  calUnit=''  calHelp=''  calAccess=1  calFunction=raptor_xcp_function(gcb)  calVisible=on
      settings: SourceProductName=Raptor
  raptor_measurement11 : Raptor_lib/Data Storage/raptor_measurement  paramName='Meas_Motor2_Actual_Speed'  nameSource=Parameter  calDispType=Number  calEnum={'False', 'True'}  calGain=1.0  calOffset=0.0  calMax=inf  calMin=-inf  calFormat='-1'  calUnit=''  calHelp=''  calAccess=1  calFunction=raptor_xcp_function(gcb)  calVisible=on
      settings: SourceProductName=Raptor
  raptor_measurement2 : Raptor_lib/Data Storage/raptor_measurement  paramName='Meas_Inverter2_Temperature'  nameSource=Parameter  calDispType=Number  calEnum={'False', 'True'}  calGain=1.0  calOffset=0.0  calMax=inf  calMin=-inf  calFormat='-1'  calUnit=''  calHelp=''  calAccess=1  calFunction=raptor_xcp_function(gcb)  calVisible=on
      settings: SourceProductName=Raptor
  raptor_measurement3 : Raptor_lib/Data Storage/raptor_measurement  paramName='Meas_Motor2_Actual_Relative_Torque'  nameSource=Parameter  calDispType=Number  calEnum={'False', 'True'}  calGain=1.0  calOffset=0.0  calMax=inf  calMin=-inf  calFormat='-1'  calUnit=''  calHelp=''  calAccess=1  calFunction=raptor_xcp_function(gcb)  calVisible=on
      settings: SourceProductName=Raptor
  raptor_measurement4 : Raptor_lib/Data Storage/raptor_measurement  paramName='Meas_Motor2_Crl_Mode'  nameSource=Parameter  calDispType=Number  calEnum={'False', 'True'}  calGain=1.0  calOffset=0.0  calMax=inf  calMin=-inf  calFormat='-1'  calUnit=''  calHelp=''  calAccess=1  calFunction=raptor_xcp_function(gcb)  calVisible=on
      settings: SourceProductName=Raptor
  raptor_measurement5 : Raptor_lib/Data Storage/raptor_measurement  paramName='Meas_Motor2_SPD_Limit'  nameSource=Parameter  calDispType=Number  calEnum={'False', 'True'}  calGain=1.0  calOffset=0.0  calMax=inf  calMin=-inf  calFormat='-1'  calUnit=''  calHelp=''  calAccess=1  calFunction=raptor_xcp_function(gcb)  calVisible=on
      settings: SourceProductName=Raptor
  raptor_measurement6 : Raptor_lib/Data Storage/raptor_measurement  paramName='Meas_Motor2_State'  nameSource=Parameter  calDispType=Number  calEnum={'False', 'True'}  calGain=1.0  calOffset=0.0  calMax=inf  calMin=-inf  calFormat='-1'  calUnit=''  calHelp=''  calAccess=1  calFunction=raptor_xcp_function(gcb)  calVisible=on
      settings: SourceProductName=Raptor
  raptor_measurement7 : Raptor_lib/Data Storage/raptor_measurement  paramName='Meas_Motor2_PWM_Output'  nameSource=Parameter  calDispType=Number  calEnum={'False', 'True'}  calGain=1.0  calOffset=0.0  calMax=inf  calMin=-inf  calFormat='-1'  calUnit=''  calHelp=''  calAccess=1  calFunction=raptor_xcp_function(gcb)  calVisible=on
      settings: SourceProductName=Raptor
  raptor_measurement8 : Raptor_lib/Data Storage/raptor_measurement  paramName='Meas_Motor2_REF_SPD_TRQ'  nameSource=Parameter  calDispType=Number  calEnum={'False', 'True'}  calGain=1.0  calOffset=0.0  calMax=inf  calMin=-inf  calFormat='-1'  calUnit=''  calHelp=''  calAccess=1  calFunction=raptor_xcp_function(gcb)  calVisible=on
      settings: SourceProductName=Raptor
  raptor_measurement9 : Raptor_lib/Data Storage/raptor_measurement  paramName='Meas_Motor2_Emergency_Stop'  nameSource=Parameter  calDispType=Number  calEnum={'False', 'True'}  calGain=1.0  calOffset=0.0  calMax=inf  calMin=-inf  calFormat='-1'  calUnit=''  calHelp=''  calAccess=1  calFunction=raptor_xcp_function(gcb)  calVisible=on
      settings: SourceProductName=Raptor
  wires:
  Constant3/1 -> Convert_Byte2Data3/1(Offset)
  Convert_Byte2Data3/1(Data) -> raptor_measurement2/1
  Constant2/1 -> Convert_Byte2Data2/1(Offset)
  Convert_Byte2Data2/1(Data) -> raptor_measurement1/1
  raptor_can_rxraw/5 -> Demux/1
  Demux/1 -> Convert_Byte2Data/1(LowByte)
  Demux/2 -> Convert_Byte2Data/2(HighByte)
  Convert_Byte2Data/1(Data) -> raptor_measurement11/1
  Convert_Byte2Data1/1(Data) -> raptor_measurement3/1
  Demux/4 -> Convert_Byte2Data1/2(HighByte)
  Demux/3 -> Convert_Byte2Data1/1(LowByte)
  Constant1/1 -> Convert_Byte2Data1/4(Factor)
  Demux/5 -> Convert_Byte2Data2/2(LowByte)
  Demux/6 -> Convert_Byte2Data3/2(LowByte)
  Demux/7 -> Byte6/1(Byte)
  Demux/8 -> Byte7/1(Byte)
  Byte6/4(Motor 2 - Emergency Stop) -> raptor_measurement9/1
  Byte6/6(Motor 2 - Speed Limit) -> raptor_measurement5/1
  Byte6/2(Motor 2 - PWM Output) -> raptor_measurement7/1
  Byte6/1(Motor 2 - Control Mode) -> raptor_measurement4/1
  Byte6/3(Motor 2 - Reference Speed/Torque) -> raptor_measurement8/1
  Byte6/5(Motor 2 - Safe Stop) -> raptor_measurement10/1
  Byte7/1(Motor 2 - State) -> raptor_measurement6/1
